simulink model "Excavator_Complete"  (R2026a)
settings: Solver=ode23t  StopTime=stopTime  MaxStep=Ts  AbsTol=1e-3
PostLoadFcn:
  | set_param(bdroot,'IgnoredZcDiagnostic','none');
  | Excavator_Test_Scenario_Select('loadedBucketDigCycle');
model workspace: external: MAT-File ExcavatorAssemblyDataStruct.mat (data not in the file)
undefined symbols (not defined in the file or in its folder): AToBRegOrificeVector, AToTOrificeVector, BiPOrificeVector, BoomC, boomHEArea, boomREArea, boomUpMaxQ, boomValve, BToTOrificeVector, BucketC, bucketCloseMaxQ, bucketOpenMaxQ, BucketR, bucketValve, fluids, gravity, LeftBoomR, materialWeight, maxPumpDisp, minPumpDisp, nominalEngineSpeed, P28Assembly, PToAOrificeVector, PToBOrificeVector, pumpCmdNegRateLimit, pumpCmdPosRateLimit, RightBoomR, startDiggingZPos, StickC, stickInMaxQ, stickOutMaxQ, StickR, stickValve, SwingC, swingDisplacement, swingHighSpeedThreshold, swingMaxQ, SwingR, swingSpeedQGain, swingValve, valveCmdNegRateLimit, valveCmdPosRateLimit, velocityToYForceGain, X, Y, yForceMax, yForceToZForceGain, Z, zForceMax
libraries: fl_lib x89, sm_lib x80, SimscapeFluids_lib x78, nesl_utility x50, simulink_extras x11, Excavator_Parts_Lib x6, simulink x2, SignalEditorBlockLib x1
(part 6 of 7)

== system Excavator_Complete/Excavator/Hydraulics/ValveBlocks/LeftValveBlock/Boom Valve ==
  AtoBRegen : SimscapeFluids_lib/Isothermal Liquid/Valves & Orifices/Orifices/Orifice (IL)  orifice_type=foundation.enum.constant_variable.variable  constant_orifice_spec=fluids.isothermal_liquid.valves_orifices.orifices.enum.constant_orifice_spec.area  variable_orifice_spec=fluids.isothermal_liquid.valves_orifices.orifices.enum.orifice_spec.table1D_area_opening  orifice_area_constant=1e-3 m^2  p_diff_TLU_constant=[-4, -3, -2, -1, -.5, 0, .5, 1, 2, 3, 4] MPa  vol_flow_TLU_constant=[-2.44, -2.12, -1.68, -1.22, -.84, 0, .85, 1.21, 1.7, 2.09, 2.41] .* 1e-3 m^3/s  S_min=1e-10 m  del_S=0.005 m  open_orientation=fluids.isothermal_liquid.valves_orifices.orifices.enum.orifice_orientation.positive  area_max=0.5e-4 m^2  area_leak=1e-12 m^2  S_TLU=valveData.spoolPosVector mm  orifice_area_TLU=valveData.AtoBRegOrificeAreaVector mm^2  area=inf m^2  Cd=0.7  Re_c=150  smoothing_factor=0  pressure_recovery=simscape.enum.onoff.off  S_vol_flow_TLU=AToBRegOrificeVector - 1000*(0) mm  p_diff_TLU=[-10000000, -5000000, -2000000, 2000000, 5000000, 10000000] Pa  vol_flow_TLU=[-1e-07, -7.0711e-08, -4.4721e-08, 4.4721e-08, 7.0711e-08, 1e-07; -2.0352e-05, -1.4391e-05, -9.1017e-06, 9.1017e-06, 1.4391e-05, 2.0352e-05; -.0040736, -.0028805, -.0018218, .0018218, .0028805, .0040736; -.011438, -.0080879, -.0051152, .0051152, .0080879, .011438; -.034356, -.024293, -.015364, .015364, .024293, .034356] m^3/s
  AtoT : SimscapeFluids_lib/Isothermal Liquid/Valves & Orifices/Orifices/Orifice (IL)  orifice_type=foundation.enum.constant_variable.variable  constant_orifice_spec=fluids.isothermal_liquid.valves_orifices.orifices.enum.constant_orifice_spec.area  variable_orifice_spec=fluids.isothermal_liquid.valves_orifices.orifices.enum.orifice_spec.table1D_area_opening  orifice_area_constant=1e-3 m^2  p_diff_TLU_constant=[-4, -3, -2, -1, -.5, 0, .5, 1, 2, 3, 4] MPa  vol_flow_TLU_constant=[-2.44, -2.12, -1.68, -1.22, -.84, 0, .85, 1.21, 1.7, 2.09, 2.41] .* 1e-3 m^3/s  S_min=1e-10 m  del_S=0.005 m  open_orientation=fluids.isothermal_liquid.valves_orifices.orifices.enum.orifice_orientation.positive  area_max=0.5e-4 m^2  area_leak=1e-12 m^2  S_TLU=valveData.spoolPosVector mm  orifice_area_TLU=valveData.AtoTOrificeAreaVector mm^2  area=inf m^2  Cd=0.7  Re_c=150  smoothing_factor=0  pressure_recovery=simscape.enum.onoff.off  S_vol_flow_TLU=AToTOrificeVector - 1000*(0) mm  p_diff_TLU=[-10000000, -5000000, -2000000, 2000000, 5000000, 10000000] Pa  vol_flow_TLU=[-1e-07, -7.0711e-08, -4.4721e-08, 4.4721e-08, 7.0711e-08, 1e-07; -2.0352e-05, -1.4391e-05, -9.1017e-06, 9.1017e-06, 1.4391e-05, 2.0352e-05; -.0040736, -.0028805, -.0018218, .0018218, .0028805, .0040736; -.011438, -.0080879, -.0051152, .0051152, .0080879, .011438; -.034356, -.024293, -.015364, .015364, .024293, .034356] m^3/s
  BiPOrifice : SimscapeFluids_lib/Isothermal Liquid/Valves & Orifices/Orifices/Orifice (IL)  orifice_type=foundation.enum.constant_variable.variable  constant_orifice_spec=fluids.isothermal_liquid.valves_orifices.orifices.enum.constant_orifice_spec.area  variable_orifice_spec=fluids.isothermal_liquid.valves_orifices.orifices.enum.orifice_spec.table1D_area_opening  orifice_area_constant=1e-3 m^2  p_diff_TLU_constant=[-4, -3, -2, -1, -.5, 0, .5, 1, 2, 3, 4] MPa  vol_flow_TLU_constant=[-2.44, -2.12, -1.68, -1.22, -.84, 0, .85, 1.21, 1.7, 2.09, 2.41] .* 1e-3 m^3/s  S_min=1e-10 m  del_S=0.005 m  open_orientation=fluids.isothermal_liquid.valves_orifices.orifices.enum.orifice_orientation.positive  area_max=0.5e-4 m^2  area_leak=1e-12 m^2  S_TLU=valveData.spoolPosVector mm  orifice_area_TLU=valveData.BiPOrificeAreaVector mm^2  area=inf m^2  Cd=0.7  Re_c=150  smoothing_factor=0  pressure_recovery=simscape.enum.onoff.off  S_vol_flow_TLU=BiPOrificeVector - 1000*(0) mm  p_diff_TLU=[-10000000, -5000000, -2000000, 2000000, 5000000, 10000000] Pa  vol_flow_TLU=[-1e-07, -7.0711e-08, -4.4721e-08, 4.4721e-08, 7.0711e-08, 1e-07; -2.0352e-05, -1.4391e-05, -9.1017e-06, 9.1017e-06, 1.4391e-05, 2.0352e-05; -.0040736, -.0028805, -.0018218, .0018218, .0028805, .0040736; -.011438, -.0080879, -.0051152, .0051152, .0080879, .011438; -.034356, -.024293, -.015364, .015364, .024293, .034356] m^3/s
  BoomRegenCV : SimscapeFluids_lib/Isothermal Liquid/Valves & Orifices/Directional Control Valves/Check Valve (IL)  opening_spec=2*(fluids.isothermal_liquid.valves_orifices.enum.opening_spec.linear)-1  pressure_control_spec=fluids.isothermal_liquid.valves_orifices.enum.pressure_control_spec.dp  p_crack_differential=valveData.checkValveCrackingPrDiff bar  p_crack_gauge=0.1 MPa  press_max_differential=valveData.checkValveMaxOpeningPrDiff bar  press_max_gauge=0.2 MPa  area_max=valveData.checkValveMaxOpeningArea mm^2  area_leak=valveData.checkValveLeakageArea mm^2  p_diff_TLU=[0.01 : 0.01 : 0.1] MPa  valve_area_TLU=[1e-10, 1e-05, 2e-05, 3e-05, 4e-05, 5e-05, 6e-05, 7.5e-05, 8.5e-05, .0001] m^2  vol_flow_TLU=[.000358, .045, .11, .191, .284, .39, .505, .63, .764, .905] .* 1e-3 m^3/s  area=inf m^2  Cd=0.7  Re_c=150  smoothing_factor=0.01  pressure_recovery=simscape.enum.onoff.off  opening_dynamics=simscape.enum.onoff.off  tau=0.1 s
  BtoT : SimscapeFluids_lib/Isothermal Liquid/Valves & Orifices/Orifices/Orifice (IL)  orifice_type=foundation.enum.constant_variable.variable  constant_orifice_spec=fluids.isothermal_liquid.valves_orifices.orifices.enum.constant_orifice_spec.area  variable_orifice_spec=fluids.isothermal_liquid.valves_orifices.orifices.enum.orifice_spec.table1D_area_opening  orifice_area_constant=1e-3 m^2  p_diff_TLU_constant=[-4, -3, -2, -1, -.5, 0, .5, 1, 2, 3, 4] MPa  vol_flow_TLU_constant=[-2.44, -2.12, -1.68, -1.22, -.84, 0, .85, 1.21, 1.7, 2.09, 2.41] .* 1e-3 m^3/s  S_min=1e-10 m  del_S=0.005 m  open_orientation=fluids.isothermal_liquid.valves_orifices.orifices.enum.orifice_orientation.positive  area_max=0.5e-4 m^2  area_leak=1e-12 m^2  S_TLU=valveData.spoolPosVector mm  orifice_area_TLU=valveData.BtoTOrificeAreaVector mm^2  area=inf m^2  Cd=0.7  Re_c=150  smoothing_factor=0  pressure_recovery=simscape.enum.onoff.off  S_vol_flow_TLU=BToTOrificeVector - 1000*(0) mm  p_diff_TLU=[-10000000, -5000000, -2000000, 2000000, 5000000, 10000000] Pa  vol_flow_TLU=[-1e-07, -7.0711e-08, -4.4721e-08, 4.4721e-08, 7.0711e-08, 1e-07; -2.0352e-05, -1.4391e-05, -9.1017e-06, 9.1017e-06, 1.4391e-05, 2.0352e-05; -.0040736, -.0028805, -.0018218, .0018218, .0028805, .0040736; -.011438, -.0080879, -.0051152, .0051152, .0080879, .011438; -.034356, -.024293, -.015364, .015364, .024293, .034356] m^3/s
  PS Abs : fl_lib/Physical Signals/Nonlinear Operators/PS Abs  ZeroCross=true
  PS Gain1 : fl_lib/Physical Signals/Functions/PS Gain  gain=-1
  PtoA : SimscapeFluids_lib/Isothermal Liquid/Valves & Orifices/Orifices/Orifice (IL)  orifice_type=foundation.enum.constant_variable.variable  constant_orifice_spec=fluids.isothermal_liquid.valves_orifices.orifices.enum.constant_orifice_spec.area  variable_orifice_spec=fluids.isothermal_liquid.valves_orifices.orifices.enum.orifice_spec.table1D_area_opening  orifice_area_constant=1e-3 m^2  p_diff_TLU_constant=[-4, -3, -2, -1, -.5, 0, .5, 1, 2, 3, 4] MPa  vol_flow_TLU_constant=[-2.44, -2.12, -1.68, -1.22, -.84, 0, .85, 1.21, 1.7, 2.09, 2.41] .* 1e-3 m^3/s  S_min=1e-10 m  del_S=0.005 m  open_orientation=fluids.isothermal_liquid.valves_orifices.orifices.enum.orifice_orientation.positive  area_max=0.5e-4 m^2  area_leak=1e-12 m^2  S_TLU=valveData.spoolPosVector mm  orifice_area_TLU=valveData.PtoAOrificeAreaVector mm^2  area=inf m^2  Cd=0.7  Re_c=150  smoothing_factor=0  pressure_recovery=simscape.enum.onoff.off  S_vol_flow_TLU=PToAOrificeVector - 1000*(0) mm  p_diff_TLU=[-10000000, -5000000, -2000000, 2000000, 5000000, 10000000] Pa  vol_flow_TLU=[-1e-07, -7.0711e-08, -4.4721e-08, 4.4721e-08, 7.0711e-08, 1e-07; -2.0352e-05, -1.4391e-05, -9.1017e-06, 9.1017e-06, 1.4391e-05, 2.0352e-05; -.0040736, -.0028805, -.0018218, .0018218, .0028805, .0040736; -.011438, -.0080879, -.0051152, .0051152, .0080879, .011438; -.034356, -.024293, -.015364, .015364, .024293, .034356] m^3/s
  PtoB : SimscapeFluids_lib/Isothermal Liquid/Valves & Orifices/Orifices/Orifice (IL)  orifice_type=foundation.enum.constant_variable.variable  constant_orifice_spec=fluids.isothermal_liquid.valves_orifices.orifices.enum.constant_orifice_spec.area  variable_orifice_spec=fluids.isothermal_liquid.valves_orifices.orifices.enum.orifice_spec.table1D_area_opening  orifice_area_constant=1e-3 m^2  p_diff_TLU_constant=[-4, -3, -2, -1, -.5, 0, .5, 1, 2, 3, 4] MPa  vol_flow_TLU_constant=[-2.44, -2.12, -1.68, -1.22, -.84, 0, .85, 1.21, 1.7, 2.09, 2.41] .* 1e-3 m^3/s  S_min=1e-10 m  del_S=0.005 m  open_orientation=fluids.isothermal_liquid.valves_orifices.orifices.enum.orifice_orientation.positive  area_max=0.5e-4 m^2  area_leak=1e-12 m^2  S_TLU=valveData.spoolPosVector mm  orifice_area_TLU=valveData.PtoBOrificeAreaVector mm^2  area=inf m^2  Cd=0.7  Re_c=150  smoothing_factor=0  pressure_recovery=simscape.enum.onoff.off  S_vol_flow_TLU=PToBOrificeVector - 1000*(0) mm  p_diff_TLU=[-10000000, -5000000, -2000000, 2000000, 5000000, 10000000] Pa  vol_flow_TLU=[-1e-07, -7.0711e-08, -4.4721e-08, 4.4721e-08, 7.0711e-08, 1e-07; -2.0352e-05, -1.4391e-05, -9.1017e-06, 9.1017e-06, 1.4391e-05, 2.0352e-05; -.0040736, -.0028805, -.0018218, .0018218, .0028805, .0040736; -.011438, -.0080879, -.0051152, .0051152, .0080879, .011438; -.034356, -.024293, -.015364, .015364, .024293, .034356] m^3/s
  Volume Regen Valve : fl_lib/Isothermal Liquid/Elements/Constant Volume Chamber (IL)  volume=vcVol m^3  p_I_specify=on  p_I_priority=High  p_I=initBoomREPr bar  p_I_nominal_specify=off  p_I_nominal_value=1  p_I_nominal_unit=MPa
  S : PMIOPort  Side=Left
  P : PMIOPort  Port=2  Side=Left
  T : PMIOPort  Port=3  Side=Left
  BiPIn : PMIOPort  Port=4  Side=Left
  A : PMIOPort  Port=5  Side=Right
  B : PMIOPort  Port=6  Side=Right
  BiPOut : PMIOPort  Port=7  Side=Right
  connections:
  BtoT/LConn2 -- PS Gain1/RConn1 -- PtoA/LConn2
  PS Abs/LConn1 -- S/RConn1 -- AtoBRegen/LConn2 -- PtoB/LConn2 -- AtoT/LConn2 -- PS Gain1/LConn1
  AtoBRegen/RConn1 -- BoomRegenCV/LConn1 -- Volume Regen Valve/LConn1
  BtoT/RConn1 -- AtoT/RConn1 -- T/RConn1
  BiPOrifice/RConn1 -- BiPOut/RConn1
  BiPOrifice/LConn1 -- BiPIn/RConn1
  AtoBRegen/LConn1 -- PtoA/RConn1 -- A/RConn1 -- AtoT/LConn1
  PtoA/LConn1 -- PtoB/LConn1 -- P/RConn1
  BtoT/LConn1 -- BoomRegenCV/RConn1 -- B/RConn1 -- PtoB/RConn1
  PS Abs/RConn1 -- BiPOrifice/LConn2

== system Excavator_Complete/Excavator/Hydraulics/ValveBlocks/LeftValveBlock/Cmd to Spool Pos ==
  Cmds : Inport
  Bus Selector : BusSelector  OutputSignals=BMSpoolPos,SKSpoolPos,SGSpoolPos
  Simulink-PS Converter : nesl_utility/Simulink-PS Converter  PhysicalDomain=network_engine_domain  SubClassName=ps_input  LeftPortType=input  RightPortType=output  PseudoPeriodic=off  Frequencies=[]  NoiseDistribution=none  NoiseParameters=[]  Unit=mm  AffineConversion=off  FilteringAndDerivatives=provide  SimscapeFilterOrder=1  InputFilterTimeConstant=0.001  UdotUserProvided=0
  Simulink-PS Converter1 : nesl_utility/Simulink-PS Converter  PhysicalDomain=network_engine_domain  SubClassName=ps_input  LeftPortType=input  RightPortType=output  PseudoPeriodic=off  Frequencies=[]  NoiseDistribution=none  NoiseParameters=[]  Unit=mm  AffineConversion=off  FilteringAndDerivatives=provide  SimscapeFilterOrder=1  InputFilterTimeConstant=0.001  UdotUserProvided=0
  Simulink-PS Converter2 : nesl_utility/Simulink-PS Converter  PhysicalDomain=network_engine_domain  SubClassName=ps_input  LeftPortType=input  RightPortType=output  PseudoPeriodic=off  Frequencies=[]  NoiseDistribution=none  NoiseParameters=[]  Unit=mm  AffineConversion=off  FilteringAndDerivatives=provide  SimscapeFilterOrder=1  InputFilterTimeConstant=0.001  UdotUserProvided=0
  BMpos : PMIOPort  Side=Right
  SKpos : PMIOPort  Port=2  Side=Right
  SGpos : PMIOPort  Port=3  Side=Right
  wires:
  Bus Selector/1 -> Simulink-PS Converter/1  "<BMSpoolPos>"
  Bus Selector/3 -> Simulink-PS Converter2/1  "<SGSpoolPos>"
  Bus Selector/2 -> Simulink-PS Converter1/1  "<SKSpoolPos>"
  Cmds/1 -> Bus Selector/1
  connections:
  Simulink-PS Converter/RConn1 -- BMpos/RConn1
  Simulink-PS Converter1/RConn1 -- SKpos/RConn1
  Simulink-PS Converter2/RConn1 -- SGpos/RConn1

== system Excavator_Complete/Excavator/Hydraulics/ValveBlocks/LeftValveBlock/Stick Valve ==
  AtoT : SimscapeFluids_lib/Isothermal Liquid/Valves & Orifices/Orifices/Orifice (IL)  orifice_type=foundation.enum.constant_variable.variable  constant_orifice_spec=fluids.isothermal_liquid.valves_orifices.orifices.enum.constant_orifice_spec.area  variable_orifice_spec=fluids.isothermal_liquid.valves_orifices.orifices.enum.orifice_spec.table1D_area_opening  orifice_area_constant=1e-3 m^2  p_diff_TLU_constant=[-4, -3, -2, -1, -.5, 0, .5, 1, 2, 3, 4] MPa  vol_flow_TLU_constant=[-2.44, -2.12, -1.68, -1.22, -.84, 0, .85, 1.21, 1.7, 2.09, 2.41] .* 1e-3 m^3/s  S_min=1e-10 m  del_S=0.005 m  open_orientation=fluids.isothermal_liquid.valves_orifices.orifices.enum.orifice_orientation.positive  area_max=0.5e-4 m^2  area_leak=1e-12 m^2  S_TLU=valveData.spoolPosVector mm  orifice_area_TLU=valveData.AtoTOrificeAreaVector mm^2  area=inf m^2  Cd=0.7  Re_c=150  smoothing_factor=0  pressure_recovery=simscape.enum.onoff.off  S_vol_flow_TLU=AToTOrificeVector - 1000*(0) mm  p_diff_TLU=[-10000000, -5000000, -2000000, 2000000, 5000000, 10000000] Pa  vol_flow_TLU=[-1e-07, -7.0711e-08, -4.4721e-08, 4.4721e-08, 7.0711e-08, 1e-07; -2.0352e-05, -1.4391e-05, -9.1017e-06, 9.1017e-06, 1.4391e-05, 2.0352e-05; -.0040736, -.0028805, -.0018218, .0018218, .0028805, .0040736; -.011438, -.0080879, -.0051152, .0051152, .0080879, .011438; -.034356, -.024293, -.015364, .015364, .024293, .034356] m^3/s
  BiPOrifice : SimscapeFluids_lib/Isothermal Liquid/Valves & Orifices/Orifices/Orifice (IL)  orifice_type=foundation.enum.constant_variable.variable  constant_orifice_spec=fluids.isothermal_liquid.valves_orifices.orifices.enum.constant_orifice_spec.area  variable_orifice_spec=fluids.isothermal_liquid.valves_orifices.orifices.enum.orifice_spec.table1D_area_opening  orifice_area_constant=1e-3 m^2  p_diff_TLU_constant=[-4, -3, -2, -1, -.5, 0, .5, 1, 2, 3, 4] MPa  vol_flow_TLU_constant=[-2.44, -2.12, -1.68, -1.22, -.84, 0, .85, 1.21, 1.7, 2.09, 2.41] .* 1e-3 m^3/s  S_min=1e-10 m  del_S=0.005 m  open_orientation=fluids.isothermal_liquid.valves_orifices.orifices.enum.orifice_orientation.positive  area_max=0.5e-4 m^2  area_leak=1e-12 m^2  S_TLU=valveData.spoolPosVector mm  orifice_area_TLU=valveData.BiPOrificeAreaVector mm^2  area=inf m^2  Cd=0.7  Re_c=150  smoothing_factor=0  pressure_recovery=simscape.enum.onoff.off  S_vol_flow_TLU=BiPOrificeVector - 1000*(0) mm  p_diff_TLU=[-10000000, -5000000, -2000000, 2000000, 5000000, 10000000] Pa  vol_flow_TLU=[-1e-07, -7.0711e-08, -4.4721e-08, 4.4721e-08, 7.0711e-08, 1e-07; -2.0352e-05, -1.4391e-05, -9.1017e-06, 9.1017e-06, 1.4391e-05, 2.0352e-05; -.0040736, -.0028805, -.0018218, .0018218, .0028805, .0040736; -.011438, -.0080879, -.0051152, .0051152, .0080879, .011438; -.034356, -.024293, -.015364, .015364, .024293, .034356] m^3/s
  BtoARegen : SimscapeFluids_lib/Isothermal Liquid/Valves & Orifices/Orifices/Orifice (IL)  orifice_type=foundation.enum.constant_variable.variable  constant_orifice_spec=fluids.isothermal_liquid.valves_orifices.orifices.enum.constant_orifice_spec.area  variable_orifice_spec=fluids.isothermal_liquid.valves_orifices.orifices.enum.orifice_spec.table1D_area_opening  orifice_area_constant=1e-3 m^2  p_diff_TLU_constant=[-4, -3, -2, -1, -.5, 0, .5, 1, 2, 3, 4] MPa  vol_flow_TLU_constant=[-2.44, -2.12, -1.68, -1.22, -.84, 0, .85, 1.21, 1.7, 2.09, 2.41] .* 1e-3 m^3/s  S_min=1e-10 m  del_S=0.005 m  open_orientation=fluids.isothermal_liquid.valves_orifices.orifices.enum.orifice_orientation.positive  area_max=0.5e-4 m^2  area_leak=1e-12 m^2  S_TLU=valveData.spoolPosVector mm  orifice_area_TLU=valveData.BtoARegOrificeAreaVector mm^2  area=inf m^2  Cd=0.7  Re_c=150  smoothing_factor=0  pressure_recovery=simscape.enum.onoff.off  S_vol_flow_TLU=AToBRegOrificeVector - 1000*(0) mm  p_diff_TLU=[-10000000, -5000000, -2000000, 2000000, 5000000, 10000000] Pa  vol_flow_TLU=[-1e-07, -7.0711e-08, -4.4721e-08, 4.4721e-08, 7.0711e-08, 1e-07; -2.0352e-05, -1.4391e-05, -9.1017e-06, 9.1017e-06, 1.4391e-05, 2.0352e-05; -.0040736, -.0028805, -.0018218, .0018218, .0028805, .0040736; -.011438, -.0080879, -.0051152, .0051152, .0080879, .011438; -.034356, -.024293, -.015364, .015364, .024293, .034356] m^3/s
  BtoT : SimscapeFluids_lib/Isothermal Liquid/Valves & Orifices/Orifices/Orifice (IL)  orifice_type=foundation.enum.constant_variable.variable  constant_orifice_spec=fluids.isothermal_liquid.valves_orifices.orifices.enum.constant_orifice_spec.area  variable_orifice_spec=fluids.isothermal_liquid.valves_orifices.orifices.enum.orifice_spec.table1D_area_opening  orifice_area_constant=1e-3 m^2  p_diff_TLU_constant=[-4, -3, -2, -1, -.5, 0, .5, 1, 2, 3, 4] MPa  vol_flow_TLU_constant=[-2.44, -2.12, -1.68, -1.22, -.84, 0, .85, 1.21, 1.7, 2.09, 2.41] .* 1e-3 m^3/s  S_min=1e-10 m  del_S=0.005 m  open_orientation=fluids.isothermal_liquid.valves_orifices.orifices.enum.orifice_orientation.positive  area_max=0.5e-4 m^2  area_leak=1e-12 m^2  S_TLU=valveData.spoolPosVector mm  orifice_area_TLU=valveData.BtoTOrificeAreaVector mm^2  area=inf m^2  Cd=0.7  Re_c=150  smoothing_factor=0  pressure_recovery=simscape.enum.onoff.off  S_vol_flow_TLU=BToTOrificeVector - 1000*(0) mm  p_diff_TLU=[-10000000, -5000000, -2000000, 2000000, 5000000, 10000000] Pa  vol_flow_TLU=[-1e-07, -7.0711e-08, -4.4721e-08, 4.4721e-08, 7.0711e-08, 1e-07; -2.0352e-05, -1.4391e-05, -9.1017e-06, 9.1017e-06, 1.4391e-05, 2.0352e-05; -.0040736, -.0028805, -.0018218, .0018218, .0028805, .0040736; -.011438, -.0080879, -.0051152, .0051152, .0080879, .011438; -.034356, -.024293, -.015364, .015364, .024293, .034356] m^3/s
  PS Abs : fl_lib/Physical Signals/Nonlinear Operators/PS Abs  ZeroCross=true
  PS Gain2 : fl_lib/Physical Signals/Functions/PS Gain  gain=-1
  PtoA : SimscapeFluids_lib/Isothermal Liquid/Valves & Orifices/Orifices/Orifice (IL)  orifice_type=foundation.enum.constant_variable.variable  constant_orifice_spec=fluids.isothermal_liquid.valves_orifices.orifices.enum.constant_orifice_spec.area  variable_orifice_spec=fluids.isothermal_liquid.valves_orifices.orifices.enum.orifice_spec.table1D_area_opening  orifice_area_constant=1e-3 m^2  p_diff_TLU_constant=[-4, -3, -2, -1, -.5, 0, .5, 1, 2, 3, 4] MPa  vol_flow_TLU_constant=[-2.44, -2.12, -1.68, -1.22, -.84, 0, .85, 1.21, 1.7, 2.09, 2.41] .* 1e-3 m^3/s  S_min=1e-10 m  del_S=0.005 m  open_orientation=fluids.isothermal_liquid.valves_orifices.orifices.enum.orifice_orientation.positive  area_max=0.5e-4 m^2  area_leak=1e-12 m^2  S_TLU=valveData.spoolPosVector mm  orifice_area_TLU=valveData.PtoAOrificeAreaVector mm^2  area=inf m^2  Cd=0.7  Re_c=150  smoothing_factor=0  pressure_recovery=simscape.enum.onoff.off  S_vol_flow_TLU=PToAOrificeVector - 1000*(0) mm  p_diff_TLU=[-10000000, -5000000, -2000000, 2000000, 5000000, 10000000] Pa  vol_flow_TLU=[-1e-07, -7.0711e-08, -4.4721e-08, 4.4721e-08, 7.0711e-08, 1e-07; -2.0352e-05, -1.4391e-05, -9.1017e-06, 9.1017e-06, 1.4391e-05, 2.0352e-05; -.0040736, -.0028805, -.0018218, .0018218, .0028805, .0040736; -.011438, -.0080879, -.0051152, .0051152, .0080879, .011438; -.034356, -.024293, -.015364, .015364, .024293, .034356] m^3/s
  PtoB : SimscapeFluids_lib/Isothermal Liquid/Valves & Orifices/Orifices/Orifice (IL)  orifice_type=foundation.enum.constant_variable.variable  constant_orifice_spec=fluids.isothermal_liquid.valves_orifices.orifices.enum.constant_orifice_spec.area  variable_orifice_spec=fluids.isothermal_liquid.valves_orifices.orifices.enum.orifice_spec.table1D_area_opening  orifice_area_constant=1e-3 m^2  p_diff_TLU_constant=[-4, -3, -2, -1, -.5, 0, .5, 1, 2, 3, 4] MPa  vol_flow_TLU_constant=[-2.44, -2.12, -1.68, -1.22, -.84, 0, .85, 1.21, 1.7, 2.09, 2.41] .* 1e-3 m^3/s  S_min=1e-10 m  del_S=0.005 m  open_orientation=fluids.isothermal_liquid.valves_orifices.orifices.enum.orifice_orientation.positive  area_max=0.5e-4 m^2  area_leak=1e-12 m^2  S_TLU=valveData.spoolPosVector mm  orifice_area_TLU=valveData.PtoBOrificeAreaVector mm^2  area=inf m^2  Cd=0.7  Re_c=150  smoothing_factor=0  pressure_recovery=simscape.enum.onoff.off  S_vol_flow_TLU=PToBOrificeVector - 1000*(0) mm  p_diff_TLU=[-10000000, -5000000, -2000000, 2000000, 5000000, 10000000] Pa  vol_flow_TLU=[-1e-07, -7.0711e-08, -4.4721e-08, 4.4721e-08, 7.0711e-08, 1e-07; -2.0352e-05, -1.4391e-05, -9.1017e-06, 9.1017e-06, 1.4391e-05, 2.0352e-05; -.0040736, -.0028805, -.0018218, .0018218, .0028805, .0040736; -.011438, -.0080879, -.0051152, .0051152, .0080879, .011438; -.034356, -.024293, -.015364, .015364, .024293, .034356] m^3/s
  StickRegenCV : SimscapeFluids_lib/Isothermal Liquid/Valves & Orifices/Directional Control Valves/Check Valve (IL)  opening_spec=2*(fluids.isothermal_liquid.valves_orifices.enum.opening_spec.linear)-1  pressure_control_spec=fluids.isothermal_liquid.valves_orifices.enum.pressure_control_spec.dp  p_crack_differential=valveData.checkValveCrackingPrDiff bar  p_crack_gauge=0.1 MPa  press_max_differential=valveData.checkValveMaxOpeningPrDiff bar  press_max_gauge=0.2 MPa  area_max=valveData.checkValveMaxOpeningArea mm^2  area_leak=valveData.checkValveLeakageArea mm^2  p_diff_TLU=[0.01 : 0.01 : 0.1] MPa  valve_area_TLU=[1e-10, 1e-05, 2e-05, 3e-05, 4e-05, 5e-05, 6e-05, 7.5e-05, 8.5e-05, .0001] m^2  vol_flow_TLU=[.000358, .045, .11, .191, .284, .39, .505, .63, .764, .905] .* 1e-3 m^3/s  area=inf m^2  Cd=0.7  Re_c=150  smoothing_factor=0.1  pressure_recovery=simscape.enum.onoff.off  opening_dynamics=simscape.enum.onoff.off  tau=0.1 s
  Volume Regen Valve : fl_lib/Isothermal Liquid/Elements/Constant Volume Chamber (IL)  volume=vcVol m^3  p_I_specify=on  p_I_priority=High  p_I=initStickHEPr bar  p_I_nominal_specify=off  p_I_nominal_value=1  p_I_nominal_unit=MPa
  S : PMIOPort  Side=Left
  P : PMIOPort  Port=2  Side=Left
  T : PMIOPort  Port=3  Side=Left
  BiPIn : PMIOPort  Port=4  Side=Left
  A : PMIOPort  Port=5  Side=Right
  B : PMIOPort  Port=6  Side=Right
  BiPOut : PMIOPort  Port=7  Side=Right
  connections:
  BtoARegen/LConn2 -- PS Gain2/RConn1 -- PtoA/LConn2 -- BtoT/LConn2
  BiPOrifice/LConn2 -- PS Abs/RConn1
  PS Gain2/LConn1 -- AtoT/LConn2 -- PtoB/LConn2 -- PS Abs/LConn1 -- S/RConn1
  BtoARegen/RConn1 -- Volume Regen Valve/LConn1 -- StickRegenCV/LConn1
  T/RConn1 -- BtoT/RConn1 -- AtoT/RConn1
  BiPOrifice/RConn1 -- BiPOut/RConn1
  BiPOrifice/LConn1 -- BiPIn/RConn1
  StickRegenCV/RConn1 -- A/RConn1 -- PtoA/RConn1 -- AtoT/LConn1
  P/RConn1 -- PtoB/LConn1 -- PtoA/LConn1
  BtoARegen/LConn1 -- PtoB/RConn1 -- BtoT/LConn1 -- B/RConn1

== system Excavator_Complete/Excavator/Hydraulics/ValveBlocks/LeftValveBlock/Swing Valve ==
  AtoT : SimscapeFluids_lib/Isothermal Liquid/Valves & Orifices/Orifices/Orifice (IL)  orifice_type=foundation.enum.constant_variable.variable  constant_orifice_spec=fluids.isothermal_liquid.valves_orifices.orifices.enum.constant_orifice_spec.area  variable_orifice_spec=fluids.isothermal_liquid.valves_orifices.orifices.enum.orifice_spec.table1D_area_opening  orifice_area_constant=1e-3 m^2  p_diff_TLU_constant=[-4, -3, -2, -1, -.5, 0, .5, 1, 2, 3, 4] MPa  vol_flow_TLU_constant=[-2.44, -2.12, -1.68, -1.22, -.84, 0, .85, 1.21, 1.7, 2.09, 2.41] .* 1e-3 m^3/s  S_min=1e-10 m  del_S=0.005 m  open_orientation=fluids.isothermal_liquid.valves_orifices.orifices.enum.orifice_orientation.positive  area_max=0.5e-4 m^2  area_leak=1e-12 m^2  S_TLU=valveData.spoolPosVector mm  orifice_area_TLU=valveData.AtoTOrificeAreaVector mm^2  area=inf m^2  Cd=0.7  Re_c=150  smoothing_factor=0  pressure_recovery=simscape.enum.onoff.off  S_vol_flow_TLU=AToTOrificeVector - 1000*(0) mm  p_diff_TLU=[-10000000, -5000000, -2000000, 2000000, 5000000, 10000000] Pa  vol_flow_TLU=[-1e-07, -7.0711e-08, -4.4721e-08, 4.4721e-08, 7.0711e-08, 1e-07; -2.0352e-05, -1.4391e-05, -9.1017e-06, 9.1017e-06, 1.4391e-05, 2.0352e-05; -.0040736, -.0028805, -.0018218, .0018218, .0028805, .0040736; -.011438, -.0080879, -.0051152, .0051152, .0080879, .011438; -.034356, -.024293, -.015364, .015364, .024293, .034356] m^3/s
  BiPOrifice : SimscapeFluids_lib/Isothermal Liquid/Valves & Orifices/Orifices/Orifice (IL)  orifice_type=foundation.enum.constant_variable.variable  constant_orifice_spec=fluids.isothermal_liquid.valves_orifices.orifices.enum.constant_orifice_spec.area  variable_orifice_spec=fluids.isothermal_liquid.valves_orifices.orifices.enum.orifice_spec.table1D_area_opening  orifice_area_constant=1e-3 m^2  p_diff_TLU_constant=[-4, -3, -2, -1, -.5, 0, .5, 1, 2, 3, 4] MPa  vol_flow_TLU_constant=[-2.44, -2.12, -1.68, -1.22, -.84, 0, .85, 1.21, 1.7, 2.09, 2.41] .* 1e-3 m^3/s  S_min=1e-10 m  del_S=0.005 m  open_orientation=fluids.isothermal_liquid.valves_orifices.orifices.enum.orifice_orientation.positive  area_max=0.5e-4 m^2  area_leak=1e-12 m^2  S_TLU=valveData.spoolPosVector mm  orifice_area_TLU=valveData.BiPOrificeAreaVector mm^2  area=inf m^2  Cd=0.7  Re_c=150  smoothing_factor=0  pressure_recovery=simscape.enum.onoff.off  S_vol_flow_TLU=BiPOrificeVector - 1000*(0) mm  p_diff_TLU=[-10000000, -5000000, -2000000, 2000000, 5000000, 10000000] Pa  vol_flow_TLU=[-1e-07, -7.0711e-08, -4.4721e-08, 4.4721e-08, 7.0711e-08, 1e-07; -2.0352e-05, -1.4391e-05, -9.1017e-06, 9.1017e-06, 1.4391e-05, 2.0352e-05; -.0040736, -.0028805, -.0018218, .0018218, .0028805, .0040736; -.011438, -.0080879, -.0051152, .0051152, .0080879, .011438; -.034356, -.024293, -.015364, .015364, .024293, .034356] m^3/s
  BtoT : SimscapeFluids_lib/Isothermal Liquid/Valves & Orifices/Orifices/Orifice (IL)  orifice_type=foundation.enum.constant_variable.variable  constant_orifice_spec=fluids.isothermal_liquid.valves_orifices.orifices.enum.constant_orifice_spec.area  variable_orifice_spec=fluids.isothermal_liquid.valves_orifices.orifices.enum.orifice_spec.table1D_area_opening  orifice_area_constant=1e-3 m^2  p_diff_TLU_constant=[-4, -3, -2, -1, -.5, 0, .5, 1, 2, 3, 4] MPa  vol_flow_TLU_constant=[-2.44, -2.12, -1.68, -1.22, -.84, 0, .85, 1.21, 1.7, 2.09, 2.41] .* 1e-3 m^3/s  S_min=1e-10 m  del_S=0.005 m  open_orientation=fluids.isothermal_liquid.valves_orifices.orifices.enum.orifice_orientation.positive  area_max=0.5e-4 m^2  area_leak=1e-12 m^2  S_TLU=valveData.spoolPosVector mm  orifice_area_TLU=valveData.BtoTOrificeAreaVector mm^2  area=inf m^2  Cd=0.7  Re_c=150  smoothing_factor=0  pressure_recovery=simscape.enum.onoff.off  S_vol_flow_TLU=BToTOrificeVector - 1000*(0) mm  p_diff_TLU=[-10000000, -5000000, -2000000, 2000000, 5000000, 10000000] Pa  vol_flow_TLU=[-1e-07, -7.0711e-08, -4.4721e-08, 4.4721e-08, 7.0711e-08, 1e-07; -2.0352e-05, -1.4391e-05, -9.1017e-06, 9.1017e-06, 1.4391e-05, 2.0352e-05; -.0040736, -.0028805, -.0018218, .0018218, .0028805, .0040736; -.011438, -.0080879, -.0051152, .0051152, .0080879, .011438; -.034356, -.024293, -.015364, .015364, .024293, .034356] m^3/s
  PS Abs : fl_lib/Physical Signals/Nonlinear Operators/PS Abs  ZeroCross=true
  PS Gain1 : fl_lib/Physical Signals/Functions/PS Gain  gain=-1
  PtoA : SimscapeFluids_lib/Isothermal Liquid/Valves & Orifices/Orifices/Orifice (IL)  orifice_type=foundation.enum.constant_variable.variable  constant_orifice_spec=fluids.isothermal_liquid.valves_orifices.orifices.enum.constant_orifice_spec.area  variable_orifice_spec=fluids.isothermal_liquid.valves_orifices.orifices.enum.orifice_spec.table1D_area_opening  orifice_area_constant=1e-3 m^2  p_diff_TLU_constant=[-4, -3, -2, -1, -.5, 0, .5, 1, 2, 3, 4] MPa  vol_flow_TLU_constant=[-2.44, -2.12, -1.68, -1.22, -.84, 0, .85, 1.21, 1.7, 2.09, 2.41] .* 1e-3 m^3/s  S_min=1e-10 m  del_S=0.005 m  open_orientation=fluids.isothermal_liquid.valves_orifices.orifices.enum.orifice_orientation.positive  area_max=0.5e-4 m^2  area_leak=1e-12 m^2  S_TLU=valveData.spoolPosVector mm  orifice_area_TLU=valveData.PtoAOrificeAreaVector mm^2  area=inf m^2  Cd=0.7  Re_c=150  smoothing_factor=0  pressure_recovery=simscape.enum.onoff.off  S_vol_flow_TLU=PToAOrificeVector - 1000*(0) mm  p_diff_TLU=[-10000000, -5000000, -2000000, 2000000, 5000000, 10000000] Pa  vol_flow_TLU=[-1e-07, -7.0711e-08, -4.4721e-08, 4.4721e-08, 7.0711e-08, 1e-07; -2.0352e-05, -1.4391e-05, -9.1017e-06, 9.1017e-06, 1.4391e-05, 2.0352e-05; -.0040736, -.0028805, -.0018218, .0018218, .0028805, .0040736; -.011438, -.0080879, -.0051152, .0051152, .0080879, .011438; -.034356, -.024293, -.015364, .015364, .024293, .034356] m^3/s
  PtoB : SimscapeFluids_lib/Isothermal Liquid/Valves & Orifices/Orifices/Orifice (IL)  orifice_type=foundation.enum.constant_variable.variable  constant_orifice_spec=fluids.isothermal_liquid.valves_orifices.orifices.enum.constant_orifice_spec.area  variable_orifice_spec=fluids.isothermal_liquid.valves_orifices.orifices.enum.orifice_spec.table1D_area_opening  orifice_area_constant=1e-3 m^2  p_diff_TLU_constant=[-4, -3, -2, -1, -.5, 0, .5, 1, 2, 3, 4] MPa  vol_flow_TLU_constant=[-2.44, -2.12, -1.68, -1.22, -.84, 0, .85, 1.21, 1.7, 2.09, 2.41] .* 1e-3 m^3/s  S_min=1e-10 m  del_S=0.005 m  open_orientation=fluids.isothermal_liquid.valves_orifices.orifices.enum.orifice_orientation.positive  area_max=0.5e-4 m^2  area_leak=1e-12 m^2  S_TLU=valveData.spoolPosVector mm  orifice_area_TLU=valveData.PtoBOrificeAreaVector mm^2  area=inf m^2  Cd=0.7  Re_c=150  smoothing_factor=0  pressure_recovery=simscape.enum.onoff.off  S_vol_flow_TLU=PToBOrificeVector - 1000*(0) mm  p_diff_TLU=[-10000000, -5000000, -2000000, 2000000, 5000000, 10000000] Pa  vol_flow_TLU=[-1e-07, -7.0711e-08, -4.4721e-08, 4.4721e-08, 7.0711e-08, 1e-07; -2.0352e-05, -1.4391e-05, -9.1017e-06, 9.1017e-06, 1.4391e-05, 2.0352e-05; -.0040736, -.0028805, -.0018218, .0018218, .0028805, .0040736; -.011438, -.0080879, -.0051152, .0051152, .0080879, .011438; -.034356, -.024293, -.015364, .015364, .024293, .034356] m^3/s
  S : PMIOPort  Side=Left
  P : PMIOPort  Port=2  Side=Left
  T : PMIOPort  Port=3  Side=Left
  BiPIn : PMIOPort  Port=4  Side=Left
  A : PMIOPort  Port=5  Side=Right
  B : PMIOPort  Port=6  Side=Right
  BiPOut : PMIOPort  Port=7  Side=Right
  connections:
  BtoT/LConn2 -- PtoA/LConn2 -- PS Gain1/RConn1
  BiPOrifice/LConn2 -- PS Abs/RConn1
  PS Gain1/LConn1 -- PtoB/LConn2 -- AtoT/LConn2 -- S/RConn1 -- PS Abs/LConn1
  BtoT/RConn1 -- T/RConn1 -- AtoT/RConn1
  BiPOrifice/RConn1 -- BiPOut/RConn1
  BiPOrifice/LConn1 -- BiPIn/RConn1
  PtoA/RConn1 -- A/RConn1 -- AtoT/LConn1
  P/RConn1 -- PtoA/LConn1 -- PtoB/LConn1
  PtoB/RConn1 -- B/RConn1 -- BtoT/LConn1

== system Excavator_Complete/Excavator/Hydraulics/ValveBlocks/RightValveBlock/Boom Valve ==
  AtoBRegen : SimscapeFluids_lib/Isothermal Liquid/Valves & Orifices/Orifices/Orifice (IL)  orifice_type=foundation.enum.constant_variable.variable  constant_orifice_spec=fluids.isothermal_liquid.valves_orifices.orifices.enum.constant_orifice_spec.area  variable_orifice_spec=fluids.isothermal_liquid.valves_orifices.orifices.enum.orifice_spec.table1D_area_opening  orifice_area_constant=1e-3 m^2  p_diff_TLU_constant=[-4, -3, -2, -1, -.5, 0, .5, 1, 2, 3, 4] MPa  vol_flow_TLU_constant=[-2.44, -2.12, -1.68, -1.22, -.84, 0, .85, 1.21, 1.7, 2.09, 2.41] .* 1e-3 m^3/s  S_min=1e-10 m  del_S=0.005 m  open_orientation=fluids.isothermal_liquid.valves_orifices.orifices.enum.orifice_orientation.positive  area_max=0.5e-4 m^2  area_leak=1e-12 m^2  S_TLU=valveData.spoolPosVector mm  orifice_area_TLU=valveData.AtoBRegOrificeAreaVector mm^2  area=inf m^2  Cd=0.7  Re_c=150  smoothing_factor=0  pressure_recovery=simscape.enum.onoff.off  S_vol_flow_TLU=AToBRegOrificeVector - 1000*(0) mm  p_diff_TLU=[-10000000, -5000000, -2000000, 2000000, 5000000, 10000000] Pa  vol_flow_TLU=[-1e-07, -7.0711e-08, -4.4721e-08, 4.4721e-08, 7.0711e-08, 1e-07; -2.0352e-05, -1.4391e-05, -9.1017e-06, 9.1017e-06, 1.4391e-05, 2.0352e-05; -.0040736, -.0028805, -.0018218, .0018218, .0028805, .0040736; -.011438, -.0080879, -.0051152, .0051152, .0080879, .011438; -.034356, -.024293, -.015364, .015364, .024293, .034356] m^3/s
  AtoT : SimscapeFluids_lib/Isothermal Liquid/Valves & Orifices/Orifices/Orifice (IL)  orifice_type=foundation.enum.constant_variable.variable  constant_orifice_spec=fluids.isothermal_liquid.valves_orifices.orifices.enum.constant_orifice_spec.area  variable_orifice_spec=fluids.isothermal_liquid.valves_orifices.orifices.enum.orifice_spec.table1D_area_opening  orifice_area_constant=1e-3 m^2  p_diff_TLU_constant=[-4, -3, -2, -1, -.5, 0, .5, 1, 2, 3, 4] MPa  vol_flow_TLU_constant=[-2.44, -2.12, -1.68, -1.22, -.84, 0, .85, 1.21, 1.7, 2.09, 2.41] .* 1e-3 m^3/s  S_min=1e-10 m  del_S=0.005 m  open_orientation=fluids.isothermal_liquid.valves_orifices.orifices.enum.orifice_orientation.positive  area_max=0.5e-4 m^2  area_leak=1e-12 m^2  S_TLU=valveData.spoolPosVector mm  orifice_area_TLU=valveData.AtoTOrificeAreaVector mm^2  area=inf m^2  Cd=0.7  Re_c=150  smoothing_factor=0  pressure_recovery=simscape.enum.onoff.off  S_vol_flow_TLU=AToTOrificeVector - 1000*(0) mm  p_diff_TLU=[-10000000, -5000000, -2000000, 2000000, 5000000, 10000000] Pa  vol_flow_TLU=[-1e-07, -7.0711e-08, -4.4721e-08, 4.4721e-08, 7.0711e-08, 1e-07; -2.0352e-05, -1.4391e-05, -9.1017e-06, 9.1017e-06, 1.4391e-05, 2.0352e-05; -.0040736, -.0028805, -.0018218, .0018218, .0028805, .0040736; -.011438, -.0080879, -.0051152, .0051152, .0080879, .011438; -.034356, -.024293, -.015364, .015364, .024293, .034356] m^3/s
  BiPOrifice : SimscapeFluids_lib/Isothermal Liquid/Valves & Orifices/Orifices/Orifice (IL)  orifice_type=foundation.enum.constant_variable.variable  constant_orifice_spec=fluids.isothermal_liquid.valves_orifices.orifices.enum.constant_orifice_spec.area  variable_orifice_spec=fluids.isothermal_liquid.valves_orifices.orifices.enum.orifice_spec.table1D_area_opening  orifice_area_constant=1e-3 m^2  p_diff_TLU_constant=[-4, -3, -2, -1, -.5, 0, .5, 1, 2, 3, 4] MPa  vol_flow_TLU_constant=[-2.44, -2.12, -1.68, -1.22, -.84, 0, .85, 1.21, 1.7, 2.09, 2.41] .* 1e-3 m^3/s  S_min=1e-10 m  del_S=0.005 m  open_orientation=fluids.isothermal_liquid.valves_orifices.orifices.enum.orifice_orientation.positive  area_max=0.5e-4 m^2  area_leak=1e-12 m^2  S_TLU=valveData.spoolPosVector mm  orifice_area_TLU=valveData.BiPOrificeAreaVector mm^2  area=inf m^2  Cd=0.7  Re_c=150  smoothing_factor=0  pressure_recovery=simscape.enum.onoff.off  S_vol_flow_TLU=BiPOrificeVector - 1000*(0) mm  p_diff_TLU=[-10000000, -5000000, -2000000, 2000000, 5000000, 10000000] Pa  vol_flow_TLU=[-1e-07, -7.0711e-08, -4.4721e-08, 4.4721e-08, 7.0711e-08, 1e-07; -2.0352e-05, -1.4391e-05, -9.1017e-06, 9.1017e-06, 1.4391e-05, 2.0352e-05; -.0040736, -.0028805, -.0018218, .0018218, .0028805, .0040736; -.011438, -.0080879, -.0051152, .0051152, .0080879, .011438; -.034356, -.024293, -.015364, .015364, .024293, .034356] m^3/s
  BoomRegenCV : SimscapeFluids_lib/Isothermal Liquid/Valves & Orifices/Directional Control Valves/Check Valve (IL)  opening_spec=2*(fluids.isothermal_liquid.valves_orifices.enum.opening_spec.linear)-1  pressure_control_spec=fluids.isothermal_liquid.valves_orifices.enum.pressure_control_spec.dp  p_crack_differential=valveData.checkValveCrackingPrDiff bar  p_crack_gauge=0.1 MPa  press_max_differential=valveData.checkValveMaxOpeningPrDiff bar  press_max_gauge=0.2 MPa  area_max=valveData.checkValveMaxOpeningArea mm^2  area_leak=valveData.checkValveLeakageArea mm^2  p_diff_TLU=[0.01 : 0.01 : 0.1] MPa  valve_area_TLU=[1e-10, 1e-05, 2e-05, 3e-05, 4e-05, 5e-05, 6e-05, 7.5e-05, 8.5e-05, .0001] m^2  vol_flow_TLU=[.000358, .045, .11, .191, .284, .39, .505, .63, .764, .905] .* 1e-3 m^3/s  area=inf m^2  Cd=0.7  Re_c=150  smoothing_factor=0.1  pressure_recovery=simscape.enum.onoff.off  opening_dynamics=simscape.enum.onoff.off  tau=0.1 s
  BtoT : SimscapeFluids_lib/Isothermal Liquid/Valves & Orifices/Orifices/Orifice (IL)  orifice_type=foundation.enum.constant_variable.variable  constant_orifice_spec=fluids.isothermal_liquid.valves_orifices.orifices.enum.constant_orifice_spec.area  variable_orifice_spec=fluids.isothermal_liquid.valves_orifices.orifices.enum.orifice_spec.table1D_area_opening  orifice_area_constant=1e-3 m^2  p_diff_TLU_constant=[-4, -3, -2, -1, -.5, 0, .5, 1, 2, 3, 4] MPa  vol_flow_TLU_constant=[-2.44, -2.12, -1.68, -1.22, -.84, 0, .85, 1.21, 1.7, 2.09, 2.41] .* 1e-3 m^3/s  S_min=1e-10 m  del_S=0.005 m  open_orientation=fluids.isothermal_liquid.valves_orifices.orifices.enum.orifice_orientation.positive  area_max=0.5e-4 m^2  area_leak=1e-12 m^2  S_TLU=valveData.spoolPosVector mm  orifice_area_TLU=valveData.BtoTOrificeAreaVector mm^2  area=inf m^2  Cd=0.7  Re_c=150  smoothing_factor=0  pressure_recovery=simscape.enum.onoff.off  S_vol_flow_TLU=BToTOrificeVector - 1000*(0) mm  p_diff_TLU=[-10000000, -5000000, -2000000, 2000000, 5000000, 10000000] Pa  vol_flow_TLU=[-1e-07, -7.0711e-08, -4.4721e-08, 4.4721e-08, 7.0711e-08, 1e-07; -2.0352e-05, -1.4391e-05, -9.1017e-06, 9.1017e-06, 1.4391e-05, 2.0352e-05; -.0040736, -.0028805, -.0018218, .0018218, .0028805, .0040736; -.011438, -.0080879, -.0051152, .0051152, .0080879, .011438; -.034356, -.024293, -.015364, .015364, .024293, .034356] m^3/s
  PS Abs : fl_lib/Physical Signals/Nonlinear Operators/PS Abs  ZeroCross=true
  PS Gain1 : fl_lib/Physical Signals/Functions/PS Gain  gain=-1
  PtoA : SimscapeFluids_lib/Isothermal Liquid/Valves & Orifices/Orifices/Orifice (IL)  orifice_type=foundation.enum.constant_variable.variable  constant_orifice_spec=fluids.isothermal_liquid.valves_orifices.orifices.enum.constant_orifice_spec.area  variable_orifice_spec=fluids.isothermal_liquid.valves_orifices.orifices.enum.orifice_spec.table1D_area_opening  orifice_area_constant=1e-3 m^2  p_diff_TLU_constant=[-4, -3, -2, -1, -.5, 0, .5, 1, 2, 3, 4] MPa  vol_flow_TLU_constant=[-2.44, -2.12, -1.68, -1.22, -.84, 0, .85, 1.21, 1.7, 2.09, 2.41] .* 1e-3 m^3/s  S_min=1e-10 m  del_S=0.005 m  open_orientation=fluids.isothermal_liquid.valves_orifices.orifices.enum.orifice_orientation.positive  area_max=0.5e-4 m^2  area_leak=1e-12 m^2  S_TLU=valveData.spoolPosVector mm  orifice_area_TLU=valveData.PtoAOrificeAreaVector mm^2  area=inf m^2  Cd=0.7  Re_c=150  smoothing_factor=0  pressure_recovery=simscape.enum.onoff.off  S_vol_flow_TLU=PToAOrificeVector - 1000*(0) mm  p_diff_TLU=[-10000000, -5000000, -2000000, 2000000, 5000000, 10000000] Pa  vol_flow_TLU=[-1e-07, -7.0711e-08, -4.4721e-08, 4.4721e-08, 7.0711e-08, 1e-07; -2.0352e-05, -1.4391e-05, -9.1017e-06, 9.1017e-06, 1.4391e-05, 2.0352e-05; -.0040736, -.0028805, -.0018218, .0018218, .0028805, .0040736; -.011438, -.0080879, -.0051152, .0051152, .0080879, .011438; -.034356, -.024293, -.015364, .015364, .024293, .034356] m^3/s
  PtoB : SimscapeFluids_lib/Isothermal Liquid/Valves & Orifices/Orifices/Orifice (IL)  orifice_type=foundation.enum.constant_variable.variable  constant_orifice_spec=fluids.isothermal_liquid.valves_orifices.orifices.enum.constant_orifice_spec.area  variable_orifice_spec=fluids.isothermal_liquid.valves_orifices.orifices.enum.orifice_spec.table1D_area_opening  orifice_area_constant=1e-3 m^2  p_diff_TLU_constant=[-4, -3, -2, -1, -.5, 0, .5, 1, 2, 3, 4] MPa  vol_flow_TLU_constant=[-2.44, -2.12, -1.68, -1.22, -.84, 0, .85, 1.21, 1.7, 2.09, 2.41] .* 1e-3 m^3/s  S_min=1e-10 m  del_S=0.005 m  open_orientation=fluids.isothermal_liquid.valves_orifices.orifices.enum.orifice_orientation.positive  area_max=0.5e-4 m^2  area_leak=1e-12 m^2  S_TLU=valveData.spoolPosVector mm  orifice_area_TLU=valveData.PtoBOrificeAreaVector mm^2  area=inf m^2  Cd=0.7  Re_c=150  smoothing_factor=0  pressure_recovery=simscape.enum.onoff.off  S_vol_flow_TLU=PToBOrificeVector - 1000*(0) mm  p_diff_TLU=[-10000000, -5000000, -2000000, 2000000, 5000000, 10000000] Pa  vol_flow_TLU=[-1e-07, -7.0711e-08, -4.4721e-08, 4.4721e-08, 7.0711e-08, 1e-07; -2.0352e-05, -1.4391e-05, -9.1017e-06, 9.1017e-06, 1.4391e-05, 2.0352e-05; -.0040736, -.0028805, -.0018218, .0018218, .0028805, .0040736; -.011438, -.0080879, -.0051152, .0051152, .0080879, .011438; -.034356, -.024293, -.015364, .015364, .024293, .034356] m^3/s
  Volume Regen Valve : fl_lib/Isothermal Liquid/Elements/Constant Volume Chamber (IL)  volume=vcVol m^3  p_I_specify=on  p_I_priority=High  p_I=initBoomREPr bar  p_I_nominal_specify=off  p_I_nominal_value=1  p_I_nominal_unit=MPa
  S : PMIOPort  Side=Left
  P : PMIOPort  Port=2  Side=Left
  T : PMIOPort  Port=3  Side=Left
  BiPIn : PMIOPort  Port=4  Side=Left
  A : PMIOPort  Port=5  Side=Right
  B : PMIOPort  Port=6  Side=Right
  BiPOut : PMIOPort  Port=7  Side=Right
  connections:
  BtoT/LConn2 -- PS Gain1/RConn1 -- PtoA/LConn2
  PS Abs/LConn1 -- S/RConn1 -- AtoT/LConn2 -- AtoBRegen/LConn2 -- PtoB/LConn2 -- PS Gain1/LConn1
  AtoBRegen/RConn1 -- Volume Regen Valve/LConn1 -- BoomRegenCV/LConn1
  BtoT/RConn1 -- AtoT/RConn1 -- T/RConn1
  BiPOrifice/RConn1 -- BiPOut/RConn1
  BiPOrifice/LConn1 -- BiPIn/RConn1
  AtoBRegen/LConn1 -- A/RConn1 -- AtoT/LConn1 -- PtoA/RConn1
  PtoA/LConn1 -- PtoB/LConn1 -- P/RConn1
  BtoT/LConn1 -- B/RConn1 -- BoomRegenCV/RConn1 -- PtoB/RConn1
  PS Abs/RConn1 -- BiPOrifice/LConn2
